simulink model "aero_radmod_dsp"  (Simulink 8.3)
settings: Solver=FixedStepDiscrete  SolverMode=SingleTasking  StartTime=0.0  StopTime=100  MaxStep=0.1  RelTol=1e-3  AbsTol=1e-6
StopFcn:
  | aero_radplot_dsp;
model workspace (MATLAB code in the model file):
  | aero_raddat_dsp;
values from neighbouring files (symbols this model uses):
  g = 32.2    [HelperGenerateRadarData.m]
  Speed = 4    [HelperGenerateRadarData.m]
  tauc = 5    [HelperGenerateRadarData.m]
  tauT = 4    [HelperGenerateRadarData.m]
undefined symbols (not defined in the file or in its folder): deltat, DiscIntNeverNeededParam
libraries: simulink x2, dspmisc x1, dspadpt3 x1
CloseFcn:
  | radarFigureHandles=findobj('type','figure');if ~isempty(radarFigureHandles);close(radarFigureHandles);end
  | clear radarFigureHandles;
  | if exist('radarLogsOut');clear radarLogsOut;end;
settings Model: Creator=The MathWorks Inc.  CovMetricSettings=d  ExtModeTrigMode=oneshot  ExtModeArmWhenConnect=off  ExtModeAutoUpdateStatusClock=off
settings DataIOCC: LimitDataPoints=off  SignalLoggingSaveFormat=Dataset  SaveOutput=off  SaveTime=off  TimeSaveName=t_sim  SignalLoggingName=radarLogsOut
settings OptimizationCC: ExpressionDepthLimit=2147483647  InitFltsAndDblsToZero=on  EfficientMapNaN2IntZero=off
settings DebuggingCC: CheckExecutionContextPreStartOutputMsg=on  CheckExecutionContextRuntimeOutputMsg=on  SignalResolutionControl=TryResolveAllWithWarning  SolverPrmCheckMsg=none  MultiTaskDSMMsg=warning  MultiTaskCondExecSysMsg=none  FcnCallInpInsideContextMsg=UseLocalSettings  StrictBusMsg=None
settings HardwareCC: TargetUnknown=on
settings RTWCC: GenerateReport=on  IncludeERTFirstTime=on

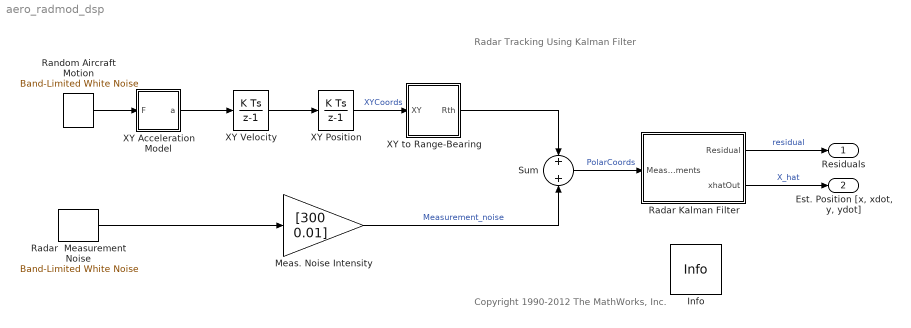
== system aero_radmod_dsp ==
  note: Copyright 1990-2012 The MathWorks, Inc.
  note: Radar Tracking Using Kalman Filter
  Info : dspmisc/Info  SystemSampleTime=-1
  Meas. Noise Intensity : Gain  Gain=[300 0.01]  SaturateOnIntegerOverflow=on  OutDataTypeStr=Inherit: Same as input  ParamDataTypeStr=Inherit: Same as input
  Radar Kalman Filter : Subsystem
  Radar  Measurement Noise : simulink/Sources/Band-Limited White Noise  Cov=[1 1]  Ts=0.1  seed=[52341 62341]
  Random Aircraft Motion : simulink/Sources/Band-Limited White Noise  Cov=[0.001 .001]  Ts=0.1  seed=[58413 74925]
  Sum : Sum  SaturateOnIntegerOverflow=on  InputSameDT=on  OutDataTypeStr=Inherit: Same as first input
  XY Acceleration Model : Subsystem
  XY Position : DiscreteIntegrator  InitialCondition=[0,Speed]  SampleTime=-1  ICPrevOutput=DiscIntNeverNeededParam  ICPrevScaledInput=DiscIntNeverNeededParam
  XY Velocity : DiscreteIntegrator  InitialCondition=[0,Speed]  SampleTime=-1  ICPrevOutput=DiscIntNeverNeededParam  ICPrevScaledInput=DiscIntNeverNeededParam
  XY to Range-Bearing : Subsystem  mask(xy2rtheta){}
      mask help:
      | Vector transformation from cartesian to polar coordinates.
      | input:   [x, y]
      | output: [r, theta]
      |
      | r = hypot(x,y));
      | theta = atan2(y,x);
      mask Help: Use "Look under mask" to see the implementation, done in Simulink blocks.
      mask Display: plot(0,0,100,100,[24,20,15,20,20],[85,95,85,95,20],[80,20,95,85,95,85],[70,20,20,15,20,24],[56,56,55,52,50,46],[20,26,31,35,38,42])
  Residuals : Outport
  "Est. Position [x, xdot, y, ydot]" : Outport  Port=2
  wires:
  Radar Kalman Filter/1(Residual) -> Residuals/1  "residual"
  Radar Kalman Filter/2(xhatOut) -> "Est. Position [x, xdot, y, ydot]"/1  "X_hat"
  Sum/1 -> Radar Kalman Filter/1(Measurements)  "PolarCoords"
  Meas. Noise Intensity/1 -> Sum/2  "Measurement_noise"
  Radar  Measurement Noise/1 -> Meas. Noise Intensity/1
  XY Acceleration Model/1(a) -> XY Velocity/1
  XY Velocity/1 -> XY Position/1
  XY Position/1 -> XY to Range-Bearing/1(XY)  "XYCoords"
  Random Aircraft Motion/1 -> XY Acceleration Model/1(F)
  XY to Range-Bearing/1(Rth) -> Sum/1

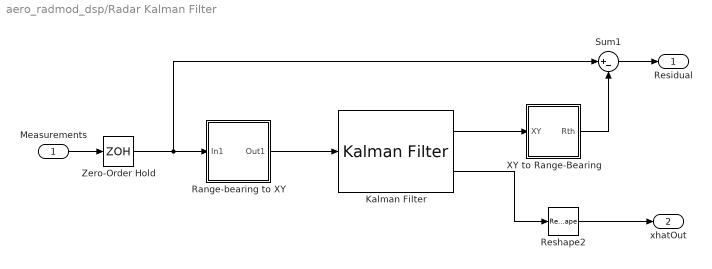
== system aero_radmod_dsp/Radar Kalman Filter ==
  Measurements : Inport
  Kalman Filter : dspadpt3/Kalman Filter  num_targets=1  sourceEnable=Always  isReset=on  X=[0.001; 0.01; 0.001; 400]  P=zeros(4)  A=[1 deltat 0 0; 0 1 0 0 ; 0 0 1 deltat; 0 0 0 1]  sourceMeasure=Specify via Dialog  H=[1 0 0 0; 0 0 1 0]  Q=diag([0 .005 0 .005])  R=300*eye(2)  isOutputEstMeasure=on  isOutputEstState=on  isOutputEstError=off  isOutputPrdMeasure=off  isOutputPrdState=off  isOutputPrdError=off
  Range-bearing to XY : Subsystem
  Reshape2 : Reshape
  Sum1 : Sum  Inputs=|+-  SaturateOnIntegerOverflow=on
  XY to Range-Bearing : Subsystem  mask(xy2rtheta){}
      mask help:
      | Vector transformation from cartesian to polar coordinates.
      | input:   [x, y]
      | output: [r, theta]
      |
      | r = hypot(x,y));
      | theta = atan2(y,x);
      mask Help: Use "Look under mask" to see the implementation, done in Simulink blocks.
      mask Display: plot(0,0,100,100,[24,20,15,20,20],[85,95,85,95,20],[80,20,95,85,95,85],[70,20,20,15,20,24],[56,56,55,52,50,46],[20,26,31,35,38,42])
  Zero-Order Hold : ZeroOrderHold  SampleTime=deltat
  Residual : Outport
  xhatOut : Outport  Port=2
  wires:
  Measurements/1 -> Zero-Order Hold/1
  Range-bearing to XY/1(Out1) -> Kalman Filter/1
  Kalman Filter/2 -> Reshape2/1
  Zero-Order Hold/1 -> Sum1/1, Range-bearing to XY/1(In1)
  Sum1/1 -> Residual/1
  Reshape2/1 -> xhatOut/1
  Kalman Filter/1 -> XY to Range-Bearing/1(XY)
  XY to Range-Bearing/1(Rth) -> Sum1/2

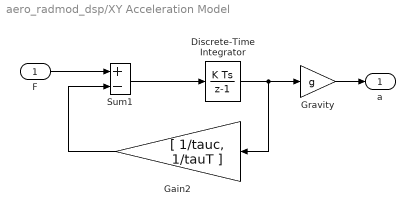
== system aero_radmod_dsp/XY Acceleration Model ==
  F : Inport
  Discrete-Time Integrator : DiscreteIntegrator  SampleTime=-1  ICPrevOutput=DiscIntNeverNeededParam  ICPrevScaledInput=DiscIntNeverNeededParam
  Gain2 : Gain  Gain=[ 1/tauc, 1/tauT ]  SaturateOnIntegerOverflow=on  OutDataTypeStr=Inherit: Same as input  ParamDataTypeStr=Inherit: Same as input
  Gravity : Gain  Gain=g  SaturateOnIntegerOverflow=on  OutDataTypeStr=Inherit: Same as input  ParamDataTypeStr=Inherit: Same as input
  Sum1 : Sum  Inputs=+-  SaturateOnIntegerOverflow=on  InputSameDT=on  OutDataTypeStr=Inherit: Same as first input
  a : Outport
  wires:
  Gravity/1 -> a/1
  Sum1/1 -> Discrete-Time Integrator/1
  Discrete-Time Integrator/1 -> Gain2/1, Gravity/1
  Gain2/1 -> Sum1/2
  F/1 -> Sum1/1

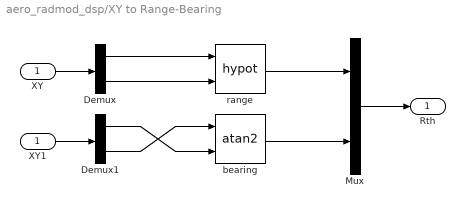
== system aero_radmod_dsp/XY to Range-Bearing ==
  XY : Inport
  Demux : Demux  Outputs=2
  Demux1 : Demux  Outputs=2
  Mux : Mux  Inputs=2
  XY1 : InportShadow
  bearing : Trigonometry  Operator=atan2
  range : Math  Operator=hypot  SaturateOnIntegerOverflow=on
  Rth : Outport  PortDimensions=2
  wires:
  Demux1/2 -> bearing/1
  Demux1/1 -> bearing/2
  bearing/1 -> Mux/2
  XY1/1 -> Demux1/1
  Demux/2 -> range/2
  Demux/1 -> range/1
  XY/1 -> Demux/1
  range/1 -> Mux/1
  Mux/1 -> Rth/1

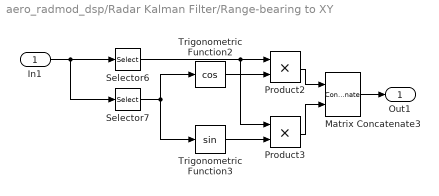
== system aero_radmod_dsp/Radar Kalman Filter/Range-bearing to XY ==
  In1 : Inport
  Matrix Concatenate3 : Concatenate  ConcatenateDimension=2
  Product2 : Product  RndMeth=Zero
  Product3 : Product  RndMeth=Zero
  Selector6 : Selector  InputPortWidth=2  Indices=[1]
  Selector7 : Selector  InputPortWidth=2  Indices=[2]
  Trigonometric Function2 : Trigonometry  Operator=cos
  Trigonometric Function3 : Trigonometry
  Out1 : Outport
  wires:
  Selector6/1 -> Product2/1, Product3/1
  Trigonometric Function2/1 -> Product2/2
  Trigonometric Function3/1 -> Product3/2
  Selector7/1 -> Trigonometric Function2/1, Trigonometric Function3/1
  Product2/1 -> Matrix Concatenate3/1
  Product3/1 -> Matrix Concatenate3/2
  In1/1 -> Selector6/1, Selector7/1
  Matrix Concatenate3/1 -> Out1/1

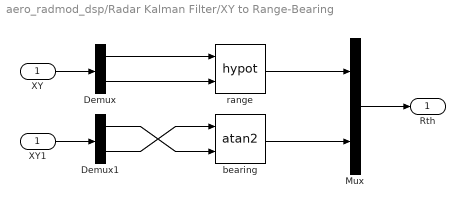
== system aero_radmod_dsp/Radar Kalman Filter/XY to Range-Bearing ==
  XY : Inport
  Demux : Demux  Outputs=2
  Demux1 : Demux  Outputs=2
  Mux : Mux  Inputs=2
  XY1 : InportShadow
  bearing : Trigonometry  Operator=atan2
  range : Math  Operator=hypot  SaturateOnIntegerOverflow=on
  Rth : Outport  PortDimensions=2
  wires:
  Mux/1 -> Rth/1
  range/1 -> Mux/1
  XY/1 -> Demux/1
  Demux/1 -> range/1
  Demux/2 -> range/2
  XY1/1 -> Demux1/1
  bearing/1 -> Mux/2
  Demux1/1 -> bearing/2
  Demux1/2 -> bearing/1
